simulink model "controlador_lazo_cerrado"  (R2019b)
settings: Solver=VariableStepAuto  StartTime=0.0  StopTime=10.0  RelTol=1e-3
values from neighbouring files (symbols this model uses):
  alfa = 2    [Lazo_abierto.m]    (also in lazo_abierto.m; lazo_cerrado.m; main.m)
  c = -12.22    [lazo_cerrado.m]
  K_c = omega_n^2 * K_g    (= 147)    [Lazo_abierto.m]    (also in lazo_abierto.m; lazo_cerrado.m = 0.0095448; main.m)
  K_g = 3    [Lazo_abierto.m]    (also in lazo_abierto.m; lazo_cerrado.m; main.m)
  omega_n = 7    [Lazo_abierto.m]    (also in lazo_abierto.m; lazo_cerrado.m; main.m)
  p = 0    [lazo_cerrado.m]
  xi = 0.5    [Lazo_abierto.m]    (also in lazo_abierto.m; lazo_cerrado.m; main.m)
settings Model: Creator=toman  LastModifiedBy=toman

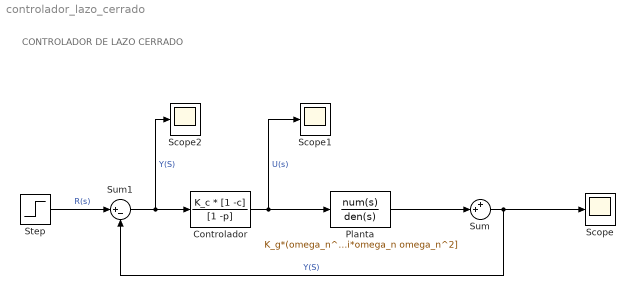
== system controlador_lazo_cerrado ==
  note: CONTROLADOR DE LAZO CERRADO
  "Controlador " : TransferFcn  Numerator=K_c * [1 -c]  Denominator=[1 -p]
  "Planta " : TransferFcn  Numerator=K_g*(omega_n^2)*[-1*alfa 1]  Denominator=[1 2*xi*omega_n omega_n^2]
  Scope : Scope
  Scope1 : Scope
  Scope2 : Scope
  Step : Step  Time=0  SampleTime=0
  Sum : Sum  Inputs=++|
  Sum1 : Sum  Inputs=|+-
  wires:
  Sum/1 -> Sum1/2, Scope/1  "Y(S)"
  "Controlador "/1 -> "Planta "/1, Scope1/1  "U(s)"
  "Planta "/1 -> Sum/2
  Step/1 -> Sum1/1  "R(s)"
  Sum1/1 -> Scope2/1, "Controlador "/1  "Y(S)"
